simulink library "INT_CrCtl_Governor"  (R2016b)
settings: Solver=VariableStepAuto  StartTime=0.0  StopTime=10.0  RelTol=1e-3
settings Model: Creator=guanxiaoxing  LastModifiedBy=guanxiaoxing

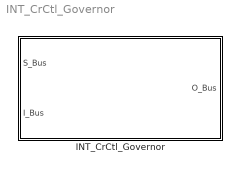
== system INT_CrCtl_Governor ==
  INT_CrCtl_Governor : Subsystem

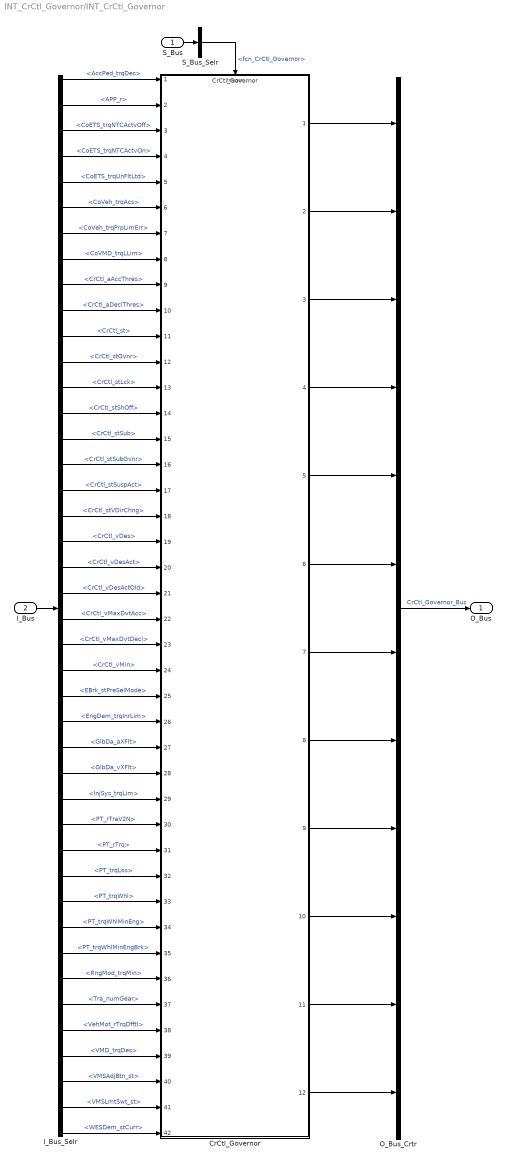
== system INT_CrCtl_Governor/INT_CrCtl_Governor ==
  S_Bus : Inport
  I_Bus : Inport  Port=2
  CrCtl_Governor : ModelReference  ModelNameDialog=CrCtl_Governor  SimulationMode=Normal  ModelReferenceVersion=1.292  TriggerPortName=function  TriggerPortTriggerType=function-call  TriggerPortStatesWhenEnabling=held
  I_Bus_Selr : BusSelector  OutputSignals=AccPed_trqDes,APP_r,CoETS_trqNTCActvOff,CoETS_trqNTCActvOn,CoETS_trqUnFltLtd,CoVeh_trqAcs,CoVeh_trqPrpLimErr,CoVMD_trqLLim,CrCtl_aAccThres,CrCtl_aDeclThres,CrCtl_st,CrCtl_stGvnr,CrCtl_stLck,CrCtl_stShOff,CrCtl_stSub,CrCtl_stSubGvnr,CrCtl_stSuspAct,CrCtl_stVDirChng,CrCtl_vDes,CrCtl_vDesAct,CrCtl_vDesActOld,CrCtl_vMaxDvtAcc,CrCtl_vMaxDvtDecl,CrCtl_vMin,EBrk_stPreSelMode,EngDem_trqInrLim,GlbDa_aXFlt,GlbDa_vXFlt,InjSys_trqLim,PT_rTraV2N,PT_rTrq,PT_trqLos,PT_trqWhl,PT_trqWhlMinEng,PT_trqWhlMinEngBrk,RngMod_trqMin,Tra_numGear,VehMot_rTrqDfftl,VMD_trqDes,VMSAdjBtn_st,VMSLmtSwt_st,WESDem_stCurr
  O_Bus_Crtr : BusCreator  Inputs=12
  S_Bus_Selr : BusSelector  OutputSignals=fcn_CrCtl_Governor
  O_Bus : Outport
  wires:
  S_Bus_Selr/1 -> CrCtl_Governor/Trigger  "<fcn_CrCtl_Governor>"
  S_Bus/1 -> S_Bus_Selr/1
  I_Bus/1 -> I_Bus_Selr/1
  I_Bus_Selr/1 -> CrCtl_Governor/1  "<AccPed_trqDes>"
  I_Bus_Selr/2 -> CrCtl_Governor/2  "<APP_r>"
  I_Bus_Selr/3 -> CrCtl_Governor/3  "<CoETS_trqNTCActvOff>"
  I_Bus_Selr/4 -> CrCtl_Governor/4  "<CoETS_trqNTCActvOn>"
  I_Bus_Selr/5 -> CrCtl_Governor/5  "<CoETS_trqUnFltLtd>"
  I_Bus_Selr/6 -> CrCtl_Governor/6  "<CoVeh_trqAcs>"
  I_Bus_Selr/7 -> CrCtl_Governor/7  "<CoVeh_trqPrpLimErr>"
  I_Bus_Selr/8 -> CrCtl_Governor/8  "<CoVMD_trqLLim>"
  I_Bus_Selr/9 -> CrCtl_Governor/9  "<CrCtl_aAccThres>"
  I_Bus_Selr/10 -> CrCtl_Governor/10  "<CrCtl_aDeclThres>"
  I_Bus_Selr/11 -> CrCtl_Governor/11  "<CrCtl_st>"
  I_Bus_Selr/12 -> CrCtl_Governor/12  "<CrCtl_stGvnr>"
  I_Bus_Selr/13 -> CrCtl_Governor/13  "<CrCtl_stLck>"
  I_Bus_Selr/14 -> CrCtl_Governor/14  "<CrCtl_stShOff>"
  I_Bus_Selr/15 -> CrCtl_Governor/15  "<CrCtl_stSub>"
  I_Bus_Selr/16 -> CrCtl_Governor/16  "<CrCtl_stSubGvnr>"
  I_Bus_Selr/17 -> CrCtl_Governor/17  "<CrCtl_stSuspAct>"
  I_Bus_Selr/18 -> CrCtl_Governor/18  "<CrCtl_stVDirChng>"
  I_Bus_Selr/19 -> CrCtl_Governor/19  "<CrCtl_vDes>"
  I_Bus_Selr/20 -> CrCtl_Governor/20  "<CrCtl_vDesAct>"
  I_Bus_Selr/21 -> CrCtl_Governor/21  "<CrCtl_vDesActOld>"
  I_Bus_Selr/22 -> CrCtl_Governor/22  "<CrCtl_vMaxDvtAcc>"
  I_Bus_Selr/23 -> CrCtl_Governor/23  "<CrCtl_vMaxDvtDecl>"
  I_Bus_Selr/24 -> CrCtl_Governor/24  "<CrCtl_vMin>"
  I_Bus_Selr/25 -> CrCtl_Governor/25  "<EBrk_stPreSelMode>"
  I_Bus_Selr/26 -> CrCtl_Governor/26  "<EngDem_trqInrLim>"
  I_Bus_Selr/27 -> CrCtl_Governor/27  "<GlbDa_aXFlt>"
  I_Bus_Selr/28 -> CrCtl_Governor/28  "<GlbDa_vXFlt>"
  I_Bus_Selr/29 -> CrCtl_Governor/29  "<InjSys_trqLim>"
  I_Bus_Selr/30 -> CrCtl_Governor/30  "<PT_rTraV2N>"
  I_Bus_Selr/31 -> CrCtl_Governor/31  "<PT_rTrq>"
  I_Bus_Selr/32 -> CrCtl_Governor/32  "<PT_trqLos>"
  I_Bus_Selr/33 -> CrCtl_Governor/33  "<PT_trqWhl>"
  I_Bus_Selr/34 -> CrCtl_Governor/34  "<PT_trqWhlMinEng>"
  I_Bus_Selr/35 -> CrCtl_Governor/35  "<PT_trqWhlMinEngBrk>"
  I_Bus_Selr/36 -> CrCtl_Governor/36  "<RngMod_trqMin>"
  I_Bus_Selr/37 -> CrCtl_Governor/37  "<Tra_numGear>"
  I_Bus_Selr/38 -> CrCtl_Governor/38  "<VehMot_rTrqDfftl>"
  I_Bus_Selr/39 -> CrCtl_Governor/39  "<VMD_trqDes>"
  I_Bus_Selr/40 -> CrCtl_Governor/40  "<VMSAdjBtn_st>"
  I_Bus_Selr/41 -> CrCtl_Governor/41  "<VMSLmtSwt_st>"
  I_Bus_Selr/42 -> CrCtl_Governor/42  "<WESDem_stCurr>"
  O_Bus_Crtr/1 -> O_Bus/1  "CrCtl_Governor_Bus"
  CrCtl_Governor/1 -> O_Bus_Crtr/1
  CrCtl_Governor/2 -> O_Bus_Crtr/2
  CrCtl_Governor/3 -> O_Bus_Crtr/3
  CrCtl_Governor/4 -> O_Bus_Crtr/4
  CrCtl_Governor/5 -> O_Bus_Crtr/5
  CrCtl_Governor/6 -> O_Bus_Crtr/6
  CrCtl_Governor/7 -> O_Bus_Crtr/7
  CrCtl_Governor/8 -> O_Bus_Crtr/8
  CrCtl_Governor/9 -> O_Bus_Crtr/9
  CrCtl_Governor/10 -> O_Bus_Crtr/10
  CrCtl_Governor/11 -> O_Bus_Crtr/11
  CrCtl_Governor/12 -> O_Bus_Crtr/12
